simulink model "QiMotorController_ModelReference"  (R2021b)
settings: Solver=FixedStepDiscrete  StartTime=0.0  StopTime=5  RelTol=1e-3
PreLoadFcn:
  | RTWConfigurationCB('preloadfcn', bdroot);
PostLoadFcn:
  | load('configuration/data_struct.mat');
  | load('configuration/fluxMaps_propMotor.mat');
  | load('configuration/parameterInit_PROP.mat');
  | load('configuration/parameterInit_PUMP.mat');
  | load('configuration/parameterInit_PITCH.mat');
  | load('configuration/parameterInit_TILT.mat');
  | %load('configuration/base_workspace_signal_definition.mat');
  | %load('resolvedatastores_to_baseworkspace_for_faster_simulation.mat');
model workspace (MAT data in the model file):
  ADC_CALIBRATION_SAMPLES : Simulink.Parameter (value not decoded)
  DEFAULT_RESOLVER_CONTROL_WORD : Simulink.Parameter (value not decoded)
  PLL_FREQUENCY : Simulink.Parameter (value not decoded)
  SIMULATION_OPTIONS : Simulink.Parameter (value not decoded)
  TARGET_CODE_GEN : Simulink.Parameter (value not decoded)
  Ts = 2.5e-07
symbols that are objects in the model workspace (value not decoded): PLL_FREQUENCY, TARGET_CODE_GEN
undefined symbols (not defined in the file): DEADTIME_NS__PITCH, DEADTIME_NS__PROP, DEADTIME_NS__PUMP, DEADTIME_NS__TILT, fIa_, fIb_, fIc_, fIdc_, fMotorEncoderFloat_, fMotorSensorSpeed_, fUa_, fUb_, fUc_, fUdc_, inbtilt, mdl_pitch_uiAPUFlags, mdl_pitch_uiFlags, modelData, oMot_, oOut_, opInputResolverData_, oPitch, oState_, PLANT_SPEED_QUADRATIC_COEFF__PUMP, POLE_PAIRS_INIT__PITCH, POLE_PAIRS_INIT__PROP, POLE_PAIRS_INIT__PUMP, POLE_PAIRS_INIT__TILT, PWM_FREQ_KHZ__PITCH, PWM_FREQ_KHZ__PROP, PWM_FREQ_KHZ__PUMP, R_PHASE_INIT__PITCH, R_PHASE_INIT__PROP, R_PHASE_INIT__TILT, R_PHASE_INIT_PLANT__PUMP, uiControlReadback_, uiGateDriverStatus_
libraries: simulink x51, spsSeriesRLCBranchLib x25, spsMosfetLib x24, powerlib_extras x24, spsCurrentMeasurementLib x17, spsVoltageMeasurementLib x17, spsPermanentMagnetSynchronousMachineLib x3, spsDCVoltageSourceLib x2, motorModelLibrary x2, slpidlib x2, cstblocks x1, spspowerguiLib x1
(part 4 of 5)

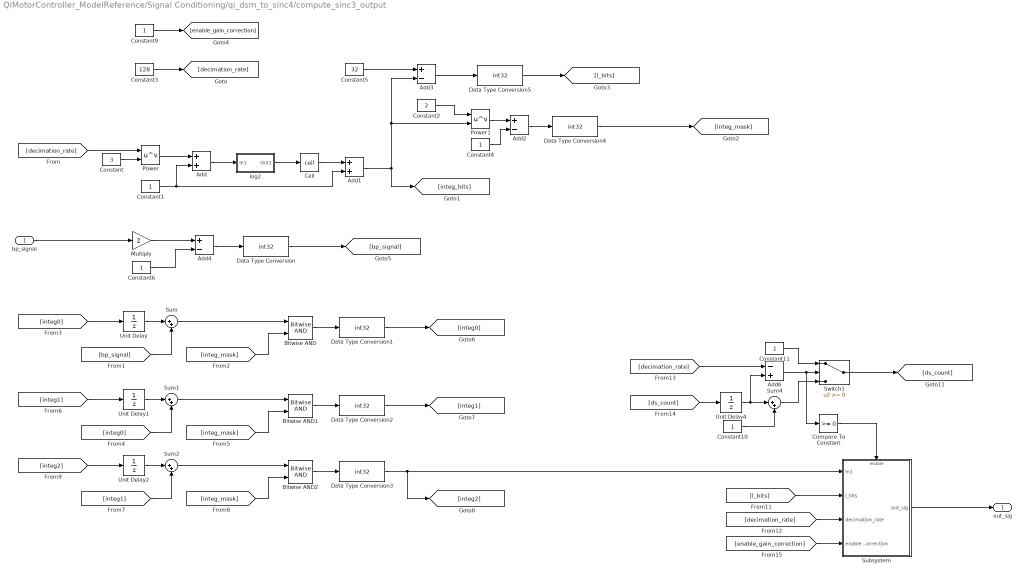
== system QiMotorController_ModelReference/Signal Conditioning/qi_dsm_to_sinc4/compute_sinc3_output ==
  bp_signal : Inport
  Add : Sum
  Add1 : Sum
  Add2 : Sum  Inputs=+-
  Add3 : Sum  Inputs=+-
  Add4 : Sum  Inputs=+-  OutDataTypeStr=int32
  Add6 : Sum  Inputs=-+  OutDataTypeStr=int32
  Bitwise AND : simulink/Logic and Bit Operations/Bitwise Operator  logicop=AND  UseBitMask=off  NumInputPorts=2  BitMask=bin2dec('11011001')  BitMaskRealWorld=Stored Integer
  Bitwise AND1 : simulink/Logic and Bit Operations/Bitwise Operator  logicop=AND  UseBitMask=off  NumInputPorts=2  BitMask=bin2dec('11011001')  BitMaskRealWorld=Stored Integer
  Bitwise AND2 : simulink/Logic and Bit Operations/Bitwise Operator  logicop=AND  UseBitMask=off  NumInputPorts=2  BitMask=bin2dec('11011001')  BitMaskRealWorld=Stored Integer
  Ceil : Rounding  Operator=ceil
  Compare To Constant : simulink/Logic and Bit Operations/Compare To Constant  relop=>=  const=0  OutDataTypeStr=boolean
  Constant : Constant  Value=3  OutDataTypeStr=single  SampleTime=-1
  Constant1 : Constant  OutDataTypeStr=single  SampleTime=-1
  Constant10 : Constant  OutDataTypeStr=int32  SampleTime=-1
  Constant11 : Constant  OutDataTypeStr=int32  SampleTime=-1
  Constant2 : Constant  Value=2  OutDataTypeStr=single  SampleTime=-1
  Constant3 : Constant  Value=128  OutDataTypeStr=single  SampleTime=-1
  Constant4 : Constant  OutDataTypeStr=single  SampleTime=-1
  Constant5 : Constant  Value=32  OutDataTypeStr=single  SampleTime=-1
  Constant6 : Constant  OutDataTypeStr=single  SampleTime=-1
  Constant9 : Constant  OutDataTypeStr=boolean  SampleTime=-1
  Data Type Conversion{,1..5} (6 alike) : DataTypeConversion  OutDataTypeStr=int32
  Multiply : Gain  Gain=2
  Power : Math  Operator=pow  SaturateOnIntegerOverflow=on
  Power1 : Math  Operator=pow  SaturateOnIntegerOverflow=on
  Subsystem : Subsystem
  Sum{,1..2,4} (4 alike) : Sum  Inputs=|++
  Switch1 : Switch
  Unit Delay : UnitDelay  SampleTime=-1  HasFrameUpgradeWarning=on
  Unit Delay1 : UnitDelay  SampleTime=-1  HasFrameUpgradeWarning=on
  Unit Delay2 : UnitDelay  SampleTime=-1  HasFrameUpgradeWarning=on
  Unit Delay4 : UnitDelay  InitialCondition=1  SampleTime=-1  HasFrameUpgradeWarning=on
  log2 : Subsystem
  out_sig : Outport
  wires:
  [decimation_rate] -> Power/1
  Constant/1 -> Power/2
  Power/1 -> Add/1
  Constant1/1 -> Add1/2, Add/2
  Constant3/1 -> [decimation_rate]
  Add/1 -> log2/1(In1)
  log2/1(Out1) -> Ceil/1
  Ceil/1 -> Add1/1
  Add1/1 -> Add3/2, Power1/2, [integ_bits]
  Constant2/1 -> Power1/1
  Power1/1 -> Add2/1
  Constant4/1 -> Add2/2
  Add2/1 -> Data Type Conversion4/1
  Constant5/1 -> Add3/1
  Add3/1 -> Data Type Conversion5/1
  bp_signal/1 -> Multiply/1
  Multiply/1 -> Add4/1
  Constant6/1 -> Add4/2
  Add4/1 -> Data Type Conversion/1
  Data Type Conversion/1 -> [bp_signal]
  Sum/1 -> Bitwise AND/1
  Unit Delay/1 -> Sum/1
  [bp_signal] -> Sum/2
  [integ_mask] -> Bitwise AND/2
  Bitwise AND/1 -> Data Type Conversion1/1
  Data Type Conversion1/1 -> [integ0]
  [integ0] -> Unit Delay/1
  Bitwise AND1/1 -> Data Type Conversion2/1
  [integ1] -> Unit Delay1/1
  [integ_mask] -> Bitwise AND1/2
  Unit Delay1/1 -> Sum1/1
  Sum1/1 -> Bitwise AND1/1
  [integ0] -> Sum1/2
  Unit Delay2/1 -> Sum2/1
  Bitwise AND2/1 -> Data Type Conversion3/1
  [integ1] -> Sum2/2
  [integ2] -> Unit Delay2/1
  Sum2/1 -> Bitwise AND2/1
  [integ_mask] -> Bitwise AND2/2
  Data Type Conversion4/1 -> [integ_mask]
  Data Type Conversion5/1 -> [l_bits]
  Constant9/1 -> [enable_gain_correction]
  Subsystem/1(out_sig) -> out_sig/1
  Sum4/1 -> Switch1/3
  Constant10/1 -> Sum4/2
  Unit Delay4/1 -> Sum4/1, Add6/2
  Constant11/1 -> Switch1/1
  Switch1/1 -> [ds_count]
  [ds_count] -> Unit Delay4/1
  [decimation_rate] -> Add6/1
  Add6/1 -> Compare To Constant/1, Switch1/2
  Compare To Constant/1 -> Subsystem/Enable
  Data Type Conversion3/1 -> [integ2], Subsystem/1(In1)
  Data Type Conversion2/1 -> [integ1]
  [l_bits] -> Subsystem/2(l_bits)
  [decimation_rate] -> Subsystem/3(decimation_rate)
  [enable_gain_correction] -> Subsystem/4(enable_gain_correction)

== system QiMotorController_ModelReference/Signal Conditioning/qi_dsm_to_sinc5/compute_dsm_output ==
  sig_in : Inport
  Add : Sum  Inputs=+-
  Add{1,3..7} (6 alike) : Sum
  Add2 : Sum  Inputs=+-
  Compare To Constant : simulink/Logic and Bit Operations/Compare To Constant  relop=>=  const=0  OutDataTypeStr=boolean
  Constant : Constant  SampleTime=-1
  Constant1 : Constant  Value=0  SampleTime=-1
  Constant2 : Constant  SampleTime=-1
  Constant3 : Constant  Value=2  SampleTime=-1
  Divide{,1..7} (8 alike) : Product  Inputs=**
  Switch : Switch  Criteria=u2 > Threshold
  Switch1 : Switch  Criteria=u2 > Threshold
  Switch2 : Switch  Criteria=u2 > Threshold
  Unit Delay{,1..6} (7 alike) : UnitDelay  SampleTime=-1  HasFrameUpgradeWarning=on
  pdm_signal : Outport
  wires:
  [b2] -> Divide/1
  [vref] -> Divide/2
  [s1_accum] -> Unit Delay1/1
  Divide/1 -> Add/2
  [s2_accum] -> Unit Delay/1
  [a2] -> Divide1/1
  Add/1 -> Divide1/2
  Unit Delay1/1 -> Add/1
  Unit Delay/1 -> Add1/1
  Divide1/1 -> Add1/2
  [vref] -> Divide2/2
  [b1] -> Divide2/1
  Divide2/1 -> Add2/2
  [a1] -> Divide3/1
  Add2/1 -> Divide3/2
  [s1_accum] -> Unit Delay2/1
  Unit Delay2/1 -> Add3/1
  Divide3/1 -> Add3/2
  [s2_accum] -> Unit Delay3/1
  Unit Delay3/1 -> Compare To Constant/1
  Add1/1 -> Switch/1
  Add3/1 -> Switch1/1
  Switch1/1 -> [s1_accum]
  Switch/1 -> [s2_accum]
  Compare To Constant/1 -> Switch1/2, Switch/2, Switch2/2
  Switch2/1 -> [dout], pdm_signal/1
  Constant/1 -> Switch2/1
  Constant1/1 -> Switch2/3
  [s2_accum] -> Unit Delay4/1
  Unit Delay4/1 -> Add5/1
  [s1_accum] -> Unit Delay5/1
  [a2] -> Divide5/1
  [vref] -> Divide4/2
  Add4/1 -> Divide5/2
  Unit Delay5/1 -> Add4/1
  [b2] -> Divide4/1
  Add5/1 -> Switch/3
  Divide5/1 -> Add5/2
  Divide4/1 -> Add4/2
  [s1_accum] -> Unit Delay6/1
  [b1] -> Divide6/1
  Divide7/1 -> Add7/2
  Add7/1 -> Switch1/3
  [a1] -> Divide7/1
  sig_in/1 -> Add6/1, Add2/1
  Add6/1 -> Divide7/2
  Unit Delay6/1 -> Add7/1
  [vref] -> Divide6/2
  Divide6/1 -> Add6/2
  Constant2/1 -> [a2], [vref], [b1], [a1]
  Constant3/1 -> [b2]

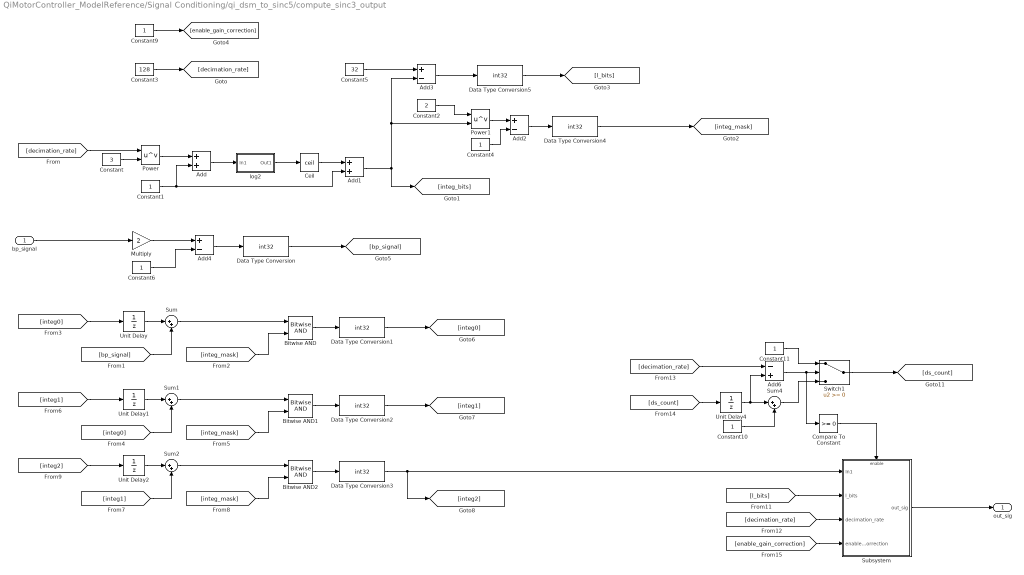
== system QiMotorController_ModelReference/Signal Conditioning/qi_dsm_to_sinc5/compute_sinc3_output ==
  bp_signal : Inport
  Add : Sum
  Add1 : Sum
  Add2 : Sum  Inputs=+-
  Add3 : Sum  Inputs=+-
  Add4 : Sum  Inputs=+-  OutDataTypeStr=int32
  Add6 : Sum  Inputs=-+  OutDataTypeStr=int32
  Bitwise AND : simulink/Logic and Bit Operations/Bitwise Operator  logicop=AND  UseBitMask=off  NumInputPorts=2  BitMask=bin2dec('11011001')  BitMaskRealWorld=Stored Integer
  Bitwise AND1 : simulink/Logic and Bit Operations/Bitwise Operator  logicop=AND  UseBitMask=off  NumInputPorts=2  BitMask=bin2dec('11011001')  BitMaskRealWorld=Stored Integer
  Bitwise AND2 : simulink/Logic and Bit Operations/Bitwise Operator  logicop=AND  UseBitMask=off  NumInputPorts=2  BitMask=bin2dec('11011001')  BitMaskRealWorld=Stored Integer
  Ceil : Rounding  Operator=ceil
  Compare To Constant : simulink/Logic and Bit Operations/Compare To Constant  relop=>=  const=0  OutDataTypeStr=boolean
  Constant : Constant  Value=3  OutDataTypeStr=single  SampleTime=-1
  Constant1 : Constant  OutDataTypeStr=single  SampleTime=-1
  Constant10 : Constant  OutDataTypeStr=int32  SampleTime=-1
  Constant11 : Constant  OutDataTypeStr=int32  SampleTime=-1
  Constant2 : Constant  Value=2  OutDataTypeStr=single  SampleTime=-1
  Constant3 : Constant  Value=128  OutDataTypeStr=single  SampleTime=-1
  Constant4 : Constant  OutDataTypeStr=single  SampleTime=-1
  Constant5 : Constant  Value=32  OutDataTypeStr=single  SampleTime=-1
  Constant6 : Constant  OutDataTypeStr=single  SampleTime=-1
  Constant9 : Constant  OutDataTypeStr=boolean  SampleTime=-1
  Data Type Conversion{,1..5} (6 alike) : DataTypeConversion  OutDataTypeStr=int32
  Multiply : Gain  Gain=2
  Power : Math  Operator=pow  SaturateOnIntegerOverflow=on
  Power1 : Math  Operator=pow  SaturateOnIntegerOverflow=on
  Subsystem : Subsystem
  Sum{,1..2,4} (4 alike) : Sum  Inputs=|++
  Switch1 : Switch
  Unit Delay : UnitDelay  SampleTime=-1  HasFrameUpgradeWarning=on
  Unit Delay1 : UnitDelay  SampleTime=-1  HasFrameUpgradeWarning=on
  Unit Delay2 : UnitDelay  SampleTime=-1  HasFrameUpgradeWarning=on
  Unit Delay4 : UnitDelay  InitialCondition=1  SampleTime=-1  HasFrameUpgradeWarning=on
  log2 : Subsystem
  out_sig : Outport
  wires:
  [decimation_rate] -> Power/1
  Constant/1 -> Power/2
  Power/1 -> Add/1
  Constant1/1 -> Add1/2, Add/2
  Constant3/1 -> [decimation_rate]
  Add/1 -> log2/1(In1)
  log2/1(Out1) -> Ceil/1
  Ceil/1 -> Add1/1
  Add1/1 -> Add3/2, Power1/2, [integ_bits]
  Constant2/1 -> Power1/1
  Power1/1 -> Add2/1
  Constant4/1 -> Add2/2
  Add2/1 -> Data Type Conversion4/1
  Constant5/1 -> Add3/1
  Add3/1 -> Data Type Conversion5/1
  bp_signal/1 -> Multiply/1
  Multiply/1 -> Add4/1
  Constant6/1 -> Add4/2
  Add4/1 -> Data Type Conversion/1
  Data Type Conversion/1 -> [bp_signal]
  Sum/1 -> Bitwise AND/1
  Unit Delay/1 -> Sum/1
  [bp_signal] -> Sum/2
  [integ_mask] -> Bitwise AND/2
  Bitwise AND/1 -> Data Type Conversion1/1
  Data Type Conversion1/1 -> [integ0]
  [integ0] -> Unit Delay/1
  Bitwise AND1/1 -> Data Type Conversion2/1
  [integ1] -> Unit Delay1/1
  [integ_mask] -> Bitwise AND1/2
  Unit Delay1/1 -> Sum1/1
  Sum1/1 -> Bitwise AND1/1
  [integ0] -> Sum1/2
  Unit Delay2/1 -> Sum2/1
  Bitwise AND2/1 -> Data Type Conversion3/1
  [integ1] -> Sum2/2
  [integ2] -> Unit Delay2/1
  Sum2/1 -> Bitwise AND2/1
  [integ_mask] -> Bitwise AND2/2
  Data Type Conversion4/1 -> [integ_mask]
  Data Type Conversion5/1 -> [l_bits]
  Constant9/1 -> [enable_gain_correction]
  Subsystem/1(out_sig) -> out_sig/1
  Sum4/1 -> Switch1/3
  Constant10/1 -> Sum4/2
  Unit Delay4/1 -> Sum4/1, Add6/2
  Constant11/1 -> Switch1/1
  Switch1/1 -> [ds_count]
  [ds_count] -> Unit Delay4/1
  [decimation_rate] -> Add6/1
  Add6/1 -> Compare To Constant/1, Switch1/2
  Compare To Constant/1 -> Subsystem/Enable
  Data Type Conversion3/1 -> [integ2], Subsystem/1(In1)
  Data Type Conversion2/1 -> [integ1]
  [l_bits] -> Subsystem/2(l_bits)
  [decimation_rate] -> Subsystem/3(decimation_rate)
  [enable_gain_correction] -> Subsystem/4(enable_gain_correction)

== system QiMotorController_ModelReference/Signal Conditioning/qi_dsm_to_sinc6/compute_dsm_output ==
  sig_in : Inport
  Add : Sum  Inputs=+-
  Add{1,3..7} (6 alike) : Sum
  Add2 : Sum  Inputs=+-
  Compare To Constant : simulink/Logic and Bit Operations/Compare To Constant  relop=>=  const=0  OutDataTypeStr=boolean
  Constant : Constant  SampleTime=-1
  Constant1 : Constant  Value=0  SampleTime=-1
  Constant2 : Constant  SampleTime=-1
  Constant3 : Constant  Value=2  SampleTime=-1
  Divide{,1..7} (8 alike) : Product  Inputs=**
  Switch : Switch  Criteria=u2 > Threshold
  Switch1 : Switch  Criteria=u2 > Threshold
  Switch2 : Switch  Criteria=u2 > Threshold
  Unit Delay{,1..6} (7 alike) : UnitDelay  SampleTime=-1  HasFrameUpgradeWarning=on
  pdm_signal : Outport
  wires:
  [b2] -> Divide/1
  [vref] -> Divide/2
  [s1_accum] -> Unit Delay1/1
  Divide/1 -> Add/2
  [s2_accum] -> Unit Delay/1
  [a2] -> Divide1/1
  Add/1 -> Divide1/2
  Unit Delay1/1 -> Add/1
  Unit Delay/1 -> Add1/1
  Divide1/1 -> Add1/2
  [vref] -> Divide2/2
  [b1] -> Divide2/1
  Divide2/1 -> Add2/2
  [a1] -> Divide3/1
  Add2/1 -> Divide3/2
  [s1_accum] -> Unit Delay2/1
  Unit Delay2/1 -> Add3/1
  Divide3/1 -> Add3/2
  [s2_accum] -> Unit Delay3/1
  Unit Delay3/1 -> Compare To Constant/1
  Add1/1 -> Switch/1
  Add3/1 -> Switch1/1
  Switch1/1 -> [s1_accum]
  Switch/1 -> [s2_accum]
  Compare To Constant/1 -> Switch1/2, Switch/2, Switch2/2
  Switch2/1 -> [dout], pdm_signal/1
  Constant/1 -> Switch2/1
  Constant1/1 -> Switch2/3
  [s2_accum] -> Unit Delay4/1
  Unit Delay4/1 -> Add5/1
  [s1_accum] -> Unit Delay5/1
  [a2] -> Divide5/1
  [vref] -> Divide4/2
  Add4/1 -> Divide5/2
  Unit Delay5/1 -> Add4/1
  [b2] -> Divide4/1
  Add5/1 -> Switch/3
  Divide5/1 -> Add5/2
  Divide4/1 -> Add4/2
  [s1_accum] -> Unit Delay6/1
  [b1] -> Divide6/1
  Divide7/1 -> Add7/2
  Add7/1 -> Switch1/3
  [a1] -> Divide7/1
  sig_in/1 -> Add6/1, Add2/1
  Add6/1 -> Divide7/2
  Unit Delay6/1 -> Add7/1
  [vref] -> Divide6/2
  Divide6/1 -> Add6/2
  Constant2/1 -> [a2], [vref], [b1], [a1]
  Constant3/1 -> [b2]

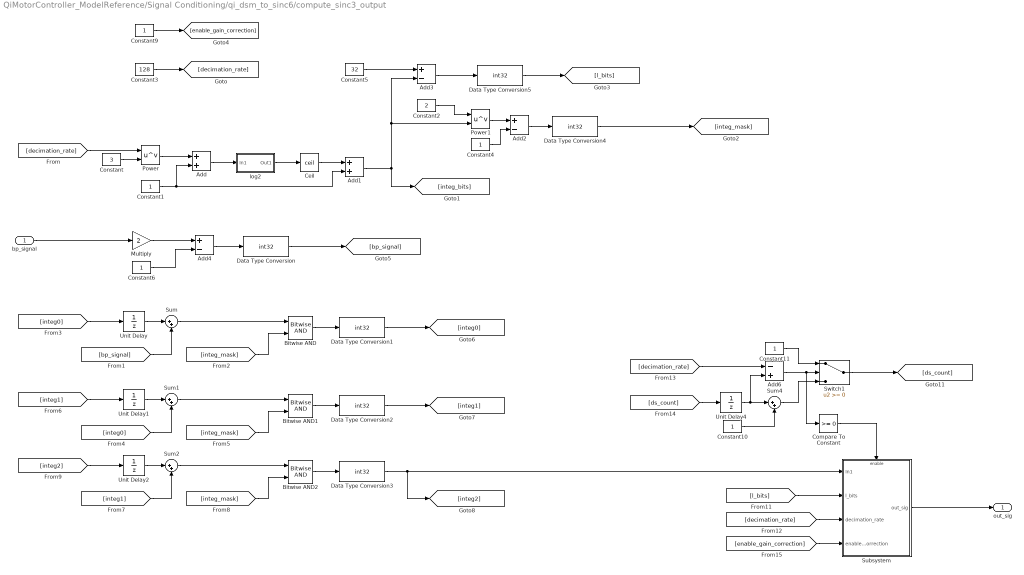
== system QiMotorController_ModelReference/Signal Conditioning/qi_dsm_to_sinc6/compute_sinc3_output ==
  bp_signal : Inport
  Add : Sum
  Add1 : Sum
  Add2 : Sum  Inputs=+-
  Add3 : Sum  Inputs=+-
  Add4 : Sum  Inputs=+-  OutDataTypeStr=int32
  Add6 : Sum  Inputs=-+  OutDataTypeStr=int32
  Bitwise AND : simulink/Logic and Bit Operations/Bitwise Operator  logicop=AND  UseBitMask=off  NumInputPorts=2  BitMask=bin2dec('11011001')  BitMaskRealWorld=Stored Integer
  Bitwise AND1 : simulink/Logic and Bit Operations/Bitwise Operator  logicop=AND  UseBitMask=off  NumInputPorts=2  BitMask=bin2dec('11011001')  BitMaskRealWorld=Stored Integer
  Bitwise AND2 : simulink/Logic and Bit Operations/Bitwise Operator  logicop=AND  UseBitMask=off  NumInputPorts=2  BitMask=bin2dec('11011001')  BitMaskRealWorld=Stored Integer
  Ceil : Rounding  Operator=ceil
  Compare To Constant : simulink/Logic and Bit Operations/Compare To Constant  relop=>=  const=0  OutDataTypeStr=boolean
  Constant : Constant  Value=3  OutDataTypeStr=single  SampleTime=-1
  Constant1 : Constant  OutDataTypeStr=single  SampleTime=-1
  Constant10 : Constant  OutDataTypeStr=int32  SampleTime=-1
  Constant11 : Constant  OutDataTypeStr=int32  SampleTime=-1
  Constant2 : Constant  Value=2  OutDataTypeStr=single  SampleTime=-1
  Constant3 : Constant  Value=128  OutDataTypeStr=single  SampleTime=-1
  Constant4 : Constant  OutDataTypeStr=single  SampleTime=-1
  Constant5 : Constant  Value=32  OutDataTypeStr=single  SampleTime=-1
  Constant6 : Constant  OutDataTypeStr=single  SampleTime=-1
  Constant9 : Constant  OutDataTypeStr=boolean  SampleTime=-1
  Data Type Conversion{,1..5} (6 alike) : DataTypeConversion  OutDataTypeStr=int32
  Multiply : Gain  Gain=2
  Power : Math  Operator=pow  SaturateOnIntegerOverflow=on
  Power1 : Math  Operator=pow  SaturateOnIntegerOverflow=on
  Subsystem : Subsystem
  Sum{,1..2,4} (4 alike) : Sum  Inputs=|++
  Switch1 : Switch
  Unit Delay : UnitDelay  SampleTime=-1  HasFrameUpgradeWarning=on
  Unit Delay1 : UnitDelay  SampleTime=-1  HasFrameUpgradeWarning=on
  Unit Delay2 : UnitDelay  SampleTime=-1  HasFrameUpgradeWarning=on
  Unit Delay4 : UnitDelay  InitialCondition=1  SampleTime=-1  HasFrameUpgradeWarning=on
  log2 : Subsystem
  out_sig : Outport
  wires:
  [decimation_rate] -> Power/1
  Constant/1 -> Power/2
  Power/1 -> Add/1
  Constant1/1 -> Add1/2, Add/2
  Constant3/1 -> [decimation_rate]
  Add/1 -> log2/1(In1)
  log2/1(Out1) -> Ceil/1
  Ceil/1 -> Add1/1
  Add1/1 -> Add3/2, Power1/2, [integ_bits]
  Constant2/1 -> Power1/1
  Power1/1 -> Add2/1
  Constant4/1 -> Add2/2
  Add2/1 -> Data Type Conversion4/1
  Constant5/1 -> Add3/1
  Add3/1 -> Data Type Conversion5/1
  bp_signal/1 -> Multiply/1
  Multiply/1 -> Add4/1
  Constant6/1 -> Add4/2
  Add4/1 -> Data Type Conversion/1
  Data Type Conversion/1 -> [bp_signal]
  Sum/1 -> Bitwise AND/1
  Unit Delay/1 -> Sum/1
  [bp_signal] -> Sum/2
  [integ_mask] -> Bitwise AND/2
  Bitwise AND/1 -> Data Type Conversion1/1
  Data Type Conversion1/1 -> [integ0]
  [integ0] -> Unit Delay/1
  Bitwise AND1/1 -> Data Type Conversion2/1
  [integ1] -> Unit Delay1/1
  [integ_mask] -> Bitwise AND1/2
  Unit Delay1/1 -> Sum1/1
  Sum1/1 -> Bitwise AND1/1
  [integ0] -> Sum1/2
  Unit Delay2/1 -> Sum2/1
  Bitwise AND2/1 -> Data Type Conversion3/1
  [integ1] -> Sum2/2
  [integ2] -> Unit Delay2/1
  Sum2/1 -> Bitwise AND2/1
  [integ_mask] -> Bitwise AND2/2
  Data Type Conversion4/1 -> [integ_mask]
  Data Type Conversion5/1 -> [l_bits]
  Constant9/1 -> [enable_gain_correction]
  Subsystem/1(out_sig) -> out_sig/1
  Sum4/1 -> Switch1/3
  Constant10/1 -> Sum4/2
  Unit Delay4/1 -> Sum4/1, Add6/2
  Constant11/1 -> Switch1/1
  Switch1/1 -> [ds_count]
  [ds_count] -> Unit Delay4/1
  [decimation_rate] -> Add6/1
  Add6/1 -> Compare To Constant/1, Switch1/2
  Compare To Constant/1 -> Subsystem/Enable
  Data Type Conversion3/1 -> [integ2], Subsystem/1(In1)
  Data Type Conversion2/1 -> [integ1]
  [l_bits] -> Subsystem/2(l_bits)
  [decimation_rate] -> Subsystem/3(decimation_rate)
  [enable_gain_correction] -> Subsystem/4(enable_gain_correction)

== system QiMotorController_ModelReference/Signal Conditioning/qi_dsm_to_sinc7/compute_dsm_output ==
  sig_in : Inport
  Add : Sum  Inputs=+-
  Add{1,3..7} (6 alike) : Sum
  Add2 : Sum  Inputs=+-
  Compare To Constant : simulink/Logic and Bit Operations/Compare To Constant  relop=>=  const=0  OutDataTypeStr=boolean
  Constant : Constant  SampleTime=-1
  Constant1 : Constant  Value=0  SampleTime=-1
  Constant2 : Constant  SampleTime=-1
  Constant3 : Constant  Value=2  SampleTime=-1
  Divide{,1..7} (8 alike) : Product  Inputs=**
  Scope : Scope  NumInputPorts=2
  Switch : Switch  Criteria=u2 > Threshold
  Switch1 : Switch  Criteria=u2 > Threshold
  Switch2 : Switch  Criteria=u2 > Threshold
  Unit Delay{,1..6} (7 alike) : UnitDelay  SampleTime=-1  HasFrameUpgradeWarning=on
  pdm_signal : Outport
  wires:
  [b2] -> Divide/1
  [vref] -> Divide/2
  [s1_accum] -> Unit Delay1/1
  Divide/1 -> Add/2
  [s2_accum] -> Unit Delay/1
  [a2] -> Divide1/1
  Add/1 -> Divide1/2
  Unit Delay1/1 -> Add/1
  Unit Delay/1 -> Add1/1
  Divide1/1 -> Add1/2
  [vref] -> Divide2/2
  [b1] -> Divide2/1
  Divide2/1 -> Add2/2
  [a1] -> Divide3/1
  Add2/1 -> Divide3/2
  [s1_accum] -> Unit Delay2/1
  Unit Delay2/1 -> Add3/1
  Divide3/1 -> Add3/2
  [s2_accum] -> Unit Delay3/1
  Unit Delay3/1 -> Compare To Constant/1
  Add1/1 -> Switch/1
  Add3/1 -> Switch1/1
  Switch1/1 -> Scope/2, [s1_accum]
  Switch/1 -> Scope/1, [s2_accum]
  Compare To Constant/1 -> Switch1/2, Switch/2, Switch2/2
  Switch2/1 -> [dout], pdm_signal/1
  Constant/1 -> Switch2/1
  Constant1/1 -> Switch2/3
  [s2_accum] -> Unit Delay4/1
  Unit Delay4/1 -> Add5/1
  [s1_accum] -> Unit Delay5/1
  [a2] -> Divide5/1
  [vref] -> Divide4/2
  Add4/1 -> Divide5/2
  Unit Delay5/1 -> Add4/1
  [b2] -> Divide4/1
  Add5/1 -> Switch/3
  Divide5/1 -> Add5/2
  Divide4/1 -> Add4/2
  [s1_accum] -> Unit Delay6/1
  [b1] -> Divide6/1
  Divide7/1 -> Add7/2
  Add7/1 -> Switch1/3
  [a1] -> Divide7/1
  sig_in/1 -> Add6/1, Add2/1
  Add6/1 -> Divide7/2
  Unit Delay6/1 -> Add7/1
  [vref] -> Divide6/2
  Divide6/1 -> Add6/2
  Constant2/1 -> [a2], [vref], [b1], [a1]
  Constant3/1 -> [b2]

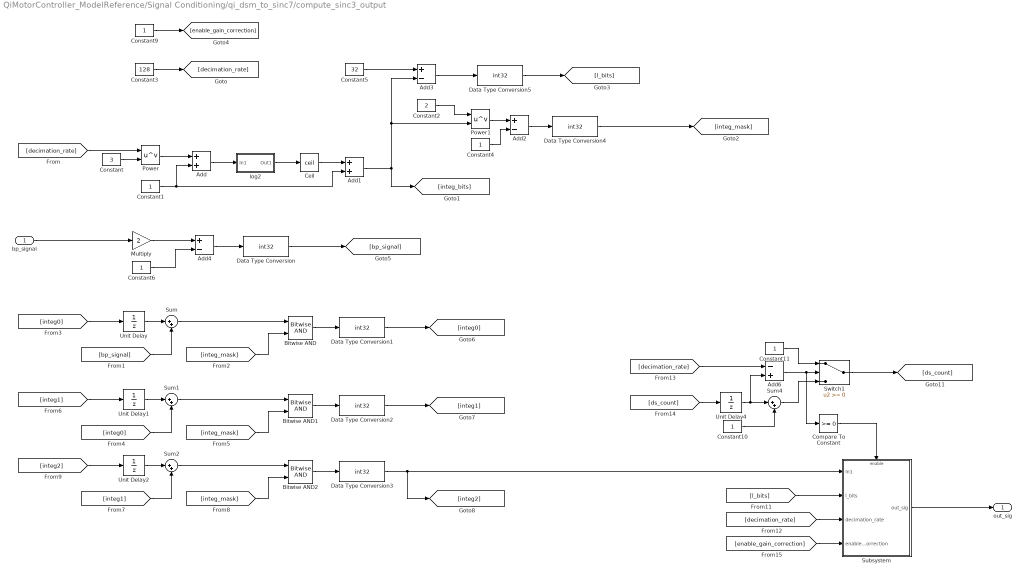
== system QiMotorController_ModelReference/Signal Conditioning/qi_dsm_to_sinc7/compute_sinc3_output ==
  bp_signal : Inport
  Add : Sum
  Add1 : Sum
  Add2 : Sum  Inputs=+-
  Add3 : Sum  Inputs=+-
  Add4 : Sum  Inputs=+-  OutDataTypeStr=int32
  Add6 : Sum  Inputs=-+  OutDataTypeStr=int32
  Bitwise AND : simulink/Logic and Bit Operations/Bitwise Operator  logicop=AND  UseBitMask=off  NumInputPorts=2  BitMask=bin2dec('11011001')  BitMaskRealWorld=Stored Integer
  Bitwise AND1 : simulink/Logic and Bit Operations/Bitwise Operator  logicop=AND  UseBitMask=off  NumInputPorts=2  BitMask=bin2dec('11011001')  BitMaskRealWorld=Stored Integer
  Bitwise AND2 : simulink/Logic and Bit Operations/Bitwise Operator  logicop=AND  UseBitMask=off  NumInputPorts=2  BitMask=bin2dec('11011001')  BitMaskRealWorld=Stored Integer
  Ceil : Rounding  Operator=ceil
  Compare To Constant : simulink/Logic and Bit Operations/Compare To Constant  relop=>=  const=0  OutDataTypeStr=boolean
  Constant : Constant  Value=3  OutDataTypeStr=single  SampleTime=-1
  Constant1 : Constant  OutDataTypeStr=single  SampleTime=-1
  Constant10 : Constant  OutDataTypeStr=int32  SampleTime=-1
  Constant11 : Constant  OutDataTypeStr=int32  SampleTime=-1
  Constant2 : Constant  Value=2  OutDataTypeStr=single  SampleTime=-1
  Constant3 : Constant  Value=128  OutDataTypeStr=single  SampleTime=-1
  Constant4 : Constant  OutDataTypeStr=single  SampleTime=-1
  Constant5 : Constant  Value=32  OutDataTypeStr=single  SampleTime=-1
  Constant6 : Constant  OutDataTypeStr=single  SampleTime=-1
  Constant9 : Constant  OutDataTypeStr=boolean  SampleTime=-1
  Data Type Conversion{,1..5} (6 alike) : DataTypeConversion  OutDataTypeStr=int32
  Multiply : Gain  Gain=2
  Power : Math  Operator=pow  SaturateOnIntegerOverflow=on
  Power1 : Math  Operator=pow  SaturateOnIntegerOverflow=on
  Subsystem : Subsystem
  Sum{,1..2,4} (4 alike) : Sum  Inputs=|++
  Switch1 : Switch
  Unit Delay : UnitDelay  SampleTime=-1  HasFrameUpgradeWarning=on
  Unit Delay1 : UnitDelay  SampleTime=-1  HasFrameUpgradeWarning=on
  Unit Delay2 : UnitDelay  SampleTime=-1  HasFrameUpgradeWarning=on
  Unit Delay4 : UnitDelay  InitialCondition=1  SampleTime=-1  HasFrameUpgradeWarning=on
  log2 : Subsystem
  out_sig : Outport
  wires:
  [decimation_rate] -> Power/1
  Constant/1 -> Power/2
  Power/1 -> Add/1
  Constant1/1 -> Add1/2, Add/2
  Constant3/1 -> [decimation_rate]
  Add/1 -> log2/1(In1)
  log2/1(Out1) -> Ceil/1
  Ceil/1 -> Add1/1
  Add1/1 -> Add3/2, Power1/2, [integ_bits]
  Constant2/1 -> Power1/1
  Power1/1 -> Add2/1
  Constant4/1 -> Add2/2
  Add2/1 -> Data Type Conversion4/1
  Constant5/1 -> Add3/1
  Add3/1 -> Data Type Conversion5/1
  bp_signal/1 -> Multiply/1
  Multiply/1 -> Add4/1
  Constant6/1 -> Add4/2
  Add4/1 -> Data Type Conversion/1
  Data Type Conversion/1 -> [bp_signal]
  Sum/1 -> Bitwise AND/1
  Unit Delay/1 -> Sum/1
  [bp_signal] -> Sum/2
  [integ_mask] -> Bitwise AND/2
  Bitwise AND/1 -> Data Type Conversion1/1
  Data Type Conversion1/1 -> [integ0]
  [integ0] -> Unit Delay/1
  Bitwise AND1/1 -> Data Type Conversion2/1
  [integ1] -> Unit Delay1/1
  [integ_mask] -> Bitwise AND1/2
  Unit Delay1/1 -> Sum1/1
  Sum1/1 -> Bitwise AND1/1
  [integ0] -> Sum1/2
  Unit Delay2/1 -> Sum2/1
  Bitwise AND2/1 -> Data Type Conversion3/1
  [integ1] -> Sum2/2
  [integ2] -> Unit Delay2/1
  Sum2/1 -> Bitwise AND2/1
  [integ_mask] -> Bitwise AND2/2
  Data Type Conversion4/1 -> [integ_mask]
  Data Type Conversion5/1 -> [l_bits]
  Constant9/1 -> [enable_gain_correction]
  Subsystem/1(out_sig) -> out_sig/1
  Sum4/1 -> Switch1/3
  Constant10/1 -> Sum4/2
  Unit Delay4/1 -> Sum4/1, Add6/2
  Constant11/1 -> Switch1/1
  Switch1/1 -> [ds_count]
  [ds_count] -> Unit Delay4/1
  [decimation_rate] -> Add6/1
  Add6/1 -> Compare To Constant/1, Switch1/2
  Compare To Constant/1 -> Subsystem/Enable
  Data Type Conversion3/1 -> [integ2], Subsystem/1(In1)
  Data Type Conversion2/1 -> [integ1]
  [l_bits] -> Subsystem/2(l_bits)
  [decimation_rate] -> Subsystem/3(decimation_rate)
  [enable_gain_correction] -> Subsystem/4(enable_gain_correction)

== system QiMotorController_ModelReference/Signal Conditioning/qi_dsm_to_sinc8/compute_dsm_output ==
  sig_in : Inport
  Add : Sum  Inputs=+-
  Add{1,3..7} (6 alike) : Sum
  Add2 : Sum  Inputs=+-
  Compare To Constant : simulink/Logic and Bit Operations/Compare To Constant  relop=>=  const=0  OutDataTypeStr=boolean
  Constant : Constant  SampleTime=-1
  Constant1 : Constant  Value=0  SampleTime=-1
  Constant2 : Constant  SampleTime=-1
  Constant3 : Constant  Value=2  SampleTime=-1
  Divide{,1..7} (8 alike) : Product  Inputs=**
  Scope : Scope  NumInputPorts=2
  Switch : Switch  Criteria=u2 > Threshold
  Switch1 : Switch  Criteria=u2 > Threshold
  Switch2 : Switch  Criteria=u2 > Threshold
  Unit Delay{,1..6} (7 alike) : UnitDelay  SampleTime=-1  HasFrameUpgradeWarning=on
  pdm_signal : Outport
  wires:
  [b2] -> Divide/1
  [vref] -> Divide/2
  [s1_accum] -> Unit Delay1/1
  Divide/1 -> Add/2
  [s2_accum] -> Unit Delay/1
  [a2] -> Divide1/1
  Add/1 -> Divide1/2
  Unit Delay1/1 -> Add/1
  Unit Delay/1 -> Add1/1
  Divide1/1 -> Add1/2
  [vref] -> Divide2/2
  [b1] -> Divide2/1
  Divide2/1 -> Add2/2
  [a1] -> Divide3/1
  Add2/1 -> Divide3/2
  [s1_accum] -> Unit Delay2/1
  Unit Delay2/1 -> Add3/1
  Divide3/1 -> Add3/2
  [s2_accum] -> Unit Delay3/1
  Unit Delay3/1 -> Compare To Constant/1
  Add1/1 -> Switch/1
  Add3/1 -> Switch1/1
  Switch1/1 -> Scope/2, [s1_accum]
  Switch/1 -> Scope/1, [s2_accum]
  Compare To Constant/1 -> Switch1/2, Switch/2, Switch2/2
  Switch2/1 -> [dout], pdm_signal/1
  Constant/1 -> Switch2/1
  Constant1/1 -> Switch2/3
  [s2_accum] -> Unit Delay4/1
  Unit Delay4/1 -> Add5/1
  [s1_accum] -> Unit Delay5/1
  [a2] -> Divide5/1
  [vref] -> Divide4/2
  Add4/1 -> Divide5/2
  Unit Delay5/1 -> Add4/1
  [b2] -> Divide4/1
  Add5/1 -> Switch/3
  Divide5/1 -> Add5/2
  Divide4/1 -> Add4/2
  [s1_accum] -> Unit Delay6/1
  [b1] -> Divide6/1
  Divide7/1 -> Add7/2
  Add7/1 -> Switch1/3
  [a1] -> Divide7/1
  sig_in/1 -> Add6/1, Add2/1
  Add6/1 -> Divide7/2
  Unit Delay6/1 -> Add7/1
  [vref] -> Divide6/2
  Divide6/1 -> Add6/2
  Constant2/1 -> [a2], [vref], [b1], [a1]
  Constant3/1 -> [b2]

== system QiMotorController_ModelReference/Signal Conditioning/qi_dsm_to_sinc8/compute_sinc3_output ==
  bp_signal : Inport
  Add : Sum
  Add1 : Sum
  Add2 : Sum  Inputs=+-
  Add3 : Sum  Inputs=+-
  Add4 : Sum  Inputs=+-  OutDataTypeStr=int32
  Add6 : Sum  Inputs=-+  OutDataTypeStr=int32
  Bitwise AND : simulink/Logic and Bit Operations/Bitwise Operator  logicop=AND  UseBitMask=off  NumInputPorts=2  BitMask=bin2dec('11011001')  BitMaskRealWorld=Stored Integer
  Bitwise AND1 : simulink/Logic and Bit Operations/Bitwise Operator  logicop=AND  UseBitMask=off  NumInputPorts=2  BitMask=bin2dec('11011001')  BitMaskRealWorld=Stored Integer
  Bitwise AND2 : simulink/Logic and Bit Operations/Bitwise Operator  logicop=AND  UseBitMask=off  NumInputPorts=2  BitMask=bin2dec('11011001')  BitMaskRealWorld=Stored Integer
  Ceil : Rounding  Operator=ceil
  Compare To Constant : simulink/Logic and Bit Operations/Compare To Constant  relop=>=  const=0  OutDataTypeStr=boolean
  Constant : Constant  Value=3  OutDataTypeStr=single  SampleTime=-1
  Constant1 : Constant  OutDataTypeStr=single  SampleTime=-1
  Constant10 : Constant  OutDataTypeStr=int32  SampleTime=-1
  Constant11 : Constant  OutDataTypeStr=int32  SampleTime=-1
  Constant2 : Constant  Value=2  OutDataTypeStr=single  SampleTime=-1
  Constant3 : Constant  Value=128  OutDataTypeStr=single  SampleTime=-1
  Constant4 : Constant  OutDataTypeStr=single  SampleTime=-1
  Constant5 : Constant  Value=32  OutDataTypeStr=single  SampleTime=-1
  Constant6 : Constant  OutDataTypeStr=single  SampleTime=-1
  Constant9 : Constant  OutDataTypeStr=boolean  SampleTime=-1
  Data Type Conversion{,1..5} (6 alike) : DataTypeConversion  OutDataTypeStr=int32
  Multiply : Gain  Gain=2
  Power : Math  Operator=pow  SaturateOnIntegerOverflow=on
  Power1 : Math  Operator=pow  SaturateOnIntegerOverflow=on
  Subsystem : Subsystem
  Sum{,1..2,4} (4 alike) : Sum  Inputs=|++
  Switch1 : Switch
  Unit Delay : UnitDelay  SampleTime=-1  HasFrameUpgradeWarning=on
  Unit Delay1 : UnitDelay  SampleTime=-1  HasFrameUpgradeWarning=on
  Unit Delay2 : UnitDelay  SampleTime=-1  HasFrameUpgradeWarning=on
  Unit Delay4 : UnitDelay  InitialCondition=1  SampleTime=-1  HasFrameUpgradeWarning=on
  log2 : Subsystem
  out_sig : Outport
  wires:
  [decimation_rate] -> Power/1
  Constant/1 -> Power/2
  Power/1 -> Add/1
  Constant1/1 -> Add1/2, Add/2
  Constant3/1 -> [decimation_rate]
  Add/1 -> log2/1(In1)
  log2/1(Out1) -> Ceil/1
  Ceil/1 -> Add1/1
  Add1/1 -> Add3/2, Power1/2, [integ_bits]
  Constant2/1 -> Power1/1
  Power1/1 -> Add2/1
  Constant4/1 -> Add2/2
  Add2/1 -> Data Type Conversion4/1
  Constant5/1 -> Add3/1
  Add3/1 -> Data Type Conversion5/1
  bp_signal/1 -> Multiply/1
  Multiply/1 -> Add4/1
  Constant6/1 -> Add4/2
  Add4/1 -> Data Type Conversion/1
  Data Type Conversion/1 -> [bp_signal]
  Sum/1 -> Bitwise AND/1
  Unit Delay/1 -> Sum/1
  [bp_signal] -> Sum/2
  [integ_mask] -> Bitwise AND/2
  Bitwise AND/1 -> Data Type Conversion1/1
  Data Type Conversion1/1 -> [integ0]
  [integ0] -> Unit Delay/1
  Bitwise AND1/1 -> Data Type Conversion2/1
  [integ1] -> Unit Delay1/1
  [integ_mask] -> Bitwise AND1/2
  Unit Delay1/1 -> Sum1/1
  Sum1/1 -> Bitwise AND1/1
  [integ0] -> Sum1/2
  Unit Delay2/1 -> Sum2/1
  Bitwise AND2/1 -> Data Type Conversion3/1
  [integ1] -> Sum2/2
  [integ2] -> Unit Delay2/1
  Sum2/1 -> Bitwise AND2/1
  [integ_mask] -> Bitwise AND2/2
  Data Type Conversion4/1 -> [integ_mask]
  Data Type Conversion5/1 -> [l_bits]
  Constant9/1 -> [enable_gain_correction]
  Subsystem/1(out_sig) -> out_sig/1
  Sum4/1 -> Switch1/3
  Constant10/1 -> Sum4/2
  Unit Delay4/1 -> Sum4/1, Add6/2
  Constant11/1 -> Switch1/1
  Switch1/1 -> [ds_count]
  [ds_count] -> Unit Delay4/1
  [decimation_rate] -> Add6/1
  Add6/1 -> Compare To Constant/1, Switch1/2
  Compare To Constant/1 -> Subsystem/Enable
  Data Type Conversion3/1 -> [integ2], Subsystem/1(In1)
  Data Type Conversion2/1 -> [integ1]
  [l_bits] -> Subsystem/2(l_bits)
  [decimation_rate] -> Subsystem/3(decimation_rate)
  [enable_gain_correction] -> Subsystem/4(enable_gain_correction)

== system QiMotorController_ModelReference/pitchMotor/PWM_pitch/Center-Aligned PWM 3-Phase   Modulator2 ==
  A_ticks : Inport
  B_ticks : Inport  Port=2
  C_ticks : Inport  Port=3
  Bias : Bias  Bias=1
  Bias1 : Bias  Bias=1
  Bias2 : Bias  Bias=1
  Gain : Gain  Gain=-1
  Gain1 : Gain  Gain=-1
  Gain2 : Gain  Gain=-1
  Mux : Mux  Inputs=6
  Rate Transition1 : RateTransition  Deterministic=off  OutPortSampleTimeOpt=Inherit  OutPortSampleTime=1/PLL_FREQUENCY
  Rate Transition2 : RateTransition  OutPortSampleTime=Ts
  Rate Transition3 : RateTransition  Deterministic=off  OutPortSampleTimeOpt=Inherit  OutPortSampleTime=1/PLL_FREQUENCY
  Rate Transition4 : RateTransition  Deterministic=off  OutPortSampleTimeOpt=Inherit  OutPortSampleTime=1/PLL_FREQUENCY
  Relay : Relay  OnSwitchValue=0  OffSwitchValue=0
  Relay1 : Relay  OnSwitchValue=0  OffSwitchValue=0
  Relay2 : Relay  OnSwitchValue=0  OffSwitchValue=0
  Repeating Sequence : simulink/Sources/Repeating Sequence  rep_seq_t=[0 1/(PWM_FREQ_KHZ__PITCH*1000)/2 1/(PWM_FREQ_KHZ__PITCH*1000)]  rep_seq_y=[0 PLL_FREQUENCY/(PWM_FREQ_KHZ__PITCH*1000)/2 0]
  Scope1 : Scope  NumInputPorts=3
  Scope2 : Scope  NumInputPorts=4
  Sum : Sum  Inputs=|+-
  Sum1 : Sum  Inputs=|+-
  Sum2 : Sum  Inputs=|+-
  PWM Gates : Outport
  wires:
  Rate Transition2/1 -> PWM Gates/1
  Mux/1 -> Rate Transition2/1
  A_ticks/1 -> Rate Transition1/1
  B_ticks/1 -> Rate Transition3/1
  C_ticks/1 -> Rate Transition4/1
  Rate Transition1/1 -> Scope2/2, Sum/1
  Rate Transition3/1 -> Scope2/3, Sum1/1
  Rate Transition4/1 -> Scope2/4, Sum2/1
  Repeating Sequence/1 -> Scope2/1, Sum/2, Sum1/2, Sum2/2
  Sum/1 -> Relay/1
  Sum2/1 -> Relay2/1
  Sum1/1 -> Relay1/1
  Relay1/1 -> Scope1/2, Mux/3, Gain1/1
  Relay2/1 -> Scope1/3, Mux/5, Gain2/1
  Gain1/1 -> Bias/1
  Gain/1 -> Bias1/1
  Gain2/1 -> Bias2/1
  Bias1/1 -> Mux/2
  Bias/1 -> Mux/4
  Bias2/1 -> Mux/6
  Relay/1 -> Gain/1, Scope1/1, Mux/1

== system QiMotorController_ModelReference/propMotor/PWM_prop/Center-Aligned PWM 3-Phase   Modulator1 ==
  Ua : Inport
  Ub : Inport  Port=2
  Uc : Inport  Port=3
  Bias : Bias  Bias=1
  Bias1 : Bias  Bias=1
  Bias2 : Bias  Bias=1
  Gain : Gain  Gain=-1
  Gain1 : Gain  Gain=-1
  Gain2 : Gain  Gain=-1
  Mux : Mux  Inputs=6
  Rate Transition1 : RateTransition  Deterministic=off  OutPortSampleTimeOpt=Inherit  OutPortSampleTime=1/PLL_FREQUENCY
  Rate Transition2 : RateTransition  OutPortSampleTime=Ts
  Rate Transition3 : RateTransition  Deterministic=off  OutPortSampleTimeOpt=Inherit  OutPortSampleTime=1/PLL_FREQUENCY
  Rate Transition4 : RateTransition  Deterministic=off  OutPortSampleTimeOpt=Inherit  OutPortSampleTime=1/PLL_FREQUENCY
  Relay : Relay  OnSwitchValue=0  OffSwitchValue=0
  Relay1 : Relay  OnSwitchValue=0  OffSwitchValue=0
  Relay2 : Relay  OnSwitchValue=0  OffSwitchValue=0
  Repeating Sequence : simulink/Sources/Repeating Sequence  rep_seq_t=[0 1/(PWM_FREQ_KHZ__PROP*1000)/2 1/(PWM_FREQ_KHZ__PROP*1000)]  rep_seq_y=[0 PLL_FREQUENCY/(PWM_FREQ_KHZ__PROP*1000)/2 0]
  Scope1 : Scope  NumInputPorts=3
  Scope2 : Scope
  Sum : Sum  Inputs=|+-
  Sum1 : Sum  Inputs=|+-
  Sum2 : Sum  Inputs=|+-
  PWM Gates : Outport
  wires:
  Rate Transition2/1 -> PWM Gates/1
  Mux/1 -> Rate Transition2/1
  Ua/1 -> Rate Transition1/1
  Ub/1 -> Rate Transition3/1
  Uc/1 -> Rate Transition4/1
  Rate Transition1/1 -> Sum/1
  Rate Transition3/1 -> Sum1/1
  Rate Transition4/1 -> Sum2/1
  Repeating Sequence/1 -> Scope2/1, Sum/2, Sum1/2, Sum2/2
  Sum/1 -> Relay/1
  Sum2/1 -> Relay2/1
  Sum1/1 -> Relay1/1
  Relay1/1 -> Scope1/2, Mux/3, Gain1/1
  Relay2/1 -> Scope1/3, Mux/5, Gain2/1
  Gain1/1 -> Bias/1
  Gain/1 -> Bias1/1
  Gain2/1 -> Bias2/1
  Bias1/1 -> Mux/2
  Bias/1 -> Mux/4
  Bias2/1 -> Mux/6
  Relay/1 -> Gain/1, Scope1/1, Mux/1

== system QiMotorController_ModelReference/propMotor/Sim Option Prop Variant Subsystem/Sim Options 0 Prop Subsystem ==
  In1 : Inport
  600 Nm torque @ 600 rpm1 : Gain  Gain=600/(600/60*2*pi)^2
  Abs1 : Abs
  Add1 : Sum
  Product3 : Product
  Sign1 : Signum
  Square1 : Math  Operator=square  SaturateOnIntegerOverflow=on
  Static friction1 : Constant  Value=10  SampleTime=-1
  Out1 : Outport
  wires:
  600 Nm torque @ 600 rpm1/1 -> Add1/2
  Square1/1 -> 600 Nm torque @ 600 rpm1/1
  Sign1/1 -> Product3/2
  Add1/1 -> Abs1/1
  In1/1 -> Sign1/1, Square1/1
  Static friction1/1 -> Add1/1
  Abs1/1 -> Product3/1
  Product3/1 -> Out1/1  "Torque"

== system QiMotorController_ModelReference/propMotor/Sim Option Prop Variant Subsystem/Sim Options 1 Prop Subsystem ==
  In1 : Inport
  Add2 : Sum  Inputs=-+|
  Constant : Constant  Value=175
  Display1 : Display
  Display2 : Display
  Gain1 : Gain  Gain=-1
  PID Controller : slpidlib/PID Controller  Controller=PI  Form=Parallel  TimeDomain=Discrete-time  UseExternalTs=off  SampleTime=-1  IntegratorMethod=Forward Euler  FilterMethod=Forward Euler  ControllerParametersSource=internal  P=500  I=10000  D=0  UseFilter=on  N=100  TunerSelectOption=Transfer Function Based (PID Tuner App)  InitialConditionSource=internal  InitialConditionForIntegrator=0  InitialConditionForFilter=0  DifferentiatorICPrevScaledInput=0  ExternalReset=none  TrackingMode=off  Kt=1  LimitOutput=on  SatLimitsSource=internal  UpperSaturationLimit=2100  LowerSaturationLimit=-2100  LinearizeAsGain=on  AntiWindupMode=clamping  Kb=1  POutMin=[]  POutMax=[]  IOutMin=[]  IOutMax=[]  DOutMin=[]  DOutMax=[]  NOutMin=[]  NOutMax=[]  SumOutMin=[]  SumOutMax=[]  SaturationOutMin=[]  SaturationOutMax=[]  PParamMin=[]  PParamMax=[]  IParamMin=[]  IParamMax=[]  DParamMin=[]  DParamMax=[]  NParamMin=[]  NParamMax=[]  KbParamMin=[]  KbParamMax=[]  KtParamMin=[]  KtParamMax=[]  KbOutMin=[]  KbOutMax=[]  KtOutMin=[]  KtOutMax=[]  IntegratorOutMin=[]  IntegratorOutMax=[]  FilterOutMin=[]  FilterOutMax=[]  SumI1OutMin=[]  SumI1OutMax=[]  SumI2OutMin=[]  SumI2OutMax=[]  SumI3OutMin=[]  SumI3OutMax=[]  SumI4OutMin=[]  SumI4OutMax=[]  SumDOutMin=[]  SumDOutMax=[]  DifferentiatorOutMin=[]  DifferentiatorOutMax=[]  FilterDiffOutCoefMin=[]  FilterDiffOutCoefMax=[]  ReciprocalOutMin=[]  ReciprocalOutMax=[]  SumDenOutMin=[]  SumDenOutMax=[]  SumNumOutMin=[]  SumNumOutMax=[]  DivideOutMin=[]  DivideOutMax=[]  UdiffTsProdOutMin=[]  UdiffTsProdOutMax=[]  NTsProdOutMin=[]  NTsProdOutMax=[]  UintegralTsProdOutMin=[]  UintegralTsProdOutMax=[]  UngainTsProdOutMin=[]  UngainTsProdOutMax=[]  IntegratorContinuousStateAttributes=''  IntegratorStateMustResolveToSignalObject=off  IntegratorRTWStateStorageClass=Auto  FilterContinuousStateAttributes=''  FilterStateMustResolveToSignalObject=off  FilterRTWStateStorageClass=Auto  ParallelPVariant=InternalParameters  IdealPVariant=Disabled  IVariant=InternalParameters  DVariant=Disabled  IntegratorVariant=Discrete  SatVariant=Enabled  AWVariant=DiscClampingParallel  PCopyVariant=Disabled  TRVariant=Disabled  FdbkBlocksVariant=Forward  IdealPFdbkVariant=Disabled  SatFdbkVariant=Disabled  DerivativeFilterVariant=Disabled  NVariant=Disabled  NCopyVariant=Disabled_SignalSpec  FilterICVariant=Disabled  IntegratorICVariant=InternalICs  ExternalResetVariant=Disabled  TRSumVariant=Passthrough  SumFdbkVariant=Disabled  SumVariant=Sum_PI  TsampFilterVariant=InternalTs  TsampNgainVariant=Passthrough  TsampIntegralVariant=Passthrough  ExternalSaturationOutDataTypeStr=Inherit: Same as second input
  RPM to rad/s2 : Gain  Gain=pi/30
  Out1 : Outport
  wires:
  PID Controller/1 -> Gain1/1
  Add2/1 -> PID Controller/1
  In1/1 -> Add2/1
  RPM to rad/s2/1 -> Display2/1, Add2/2
  Gain1/1 -> Out1/1, Display1/1
  Constant/1 -> RPM to rad/s2/1

== system QiMotorController_ModelReference/pumpfanMotor/PWM_pumpfan/Center-Aligned PWM 3-Phase   Modulator1 ==
  Ua : Inport
  Ub : Inport  Port=2
  Uc : Inport  Port=3
  Bias : Bias  Bias=1
  Bias1 : Bias  Bias=1
  Bias2 : Bias  Bias=1
  Gain : Gain  Gain=-1
  Gain1 : Gain  Gain=-1
  Gain2 : Gain  Gain=-1
  Mux : Mux  Inputs=6
  Rate Transition1 : RateTransition  Deterministic=off  OutPortSampleTimeOpt=Inherit  OutPortSampleTime=1/PLL_FREQUENCY
  Rate Transition2 : RateTransition  OutPortSampleTime=Ts
  Rate Transition3 : RateTransition  Deterministic=off  OutPortSampleTimeOpt=Inherit  OutPortSampleTime=1/PLL_FREQUENCY
  Rate Transition4 : RateTransition  Deterministic=off  OutPortSampleTimeOpt=Inherit  OutPortSampleTime=1/PLL_FREQUENCY
  Relay : Relay  OnSwitchValue=0  OffSwitchValue=0
  Relay1 : Relay  OnSwitchValue=0  OffSwitchValue=0
  Relay2 : Relay  OnSwitchValue=0  OffSwitchValue=0
  Repeating Sequence : simulink/Sources/Repeating Sequence  rep_seq_t=[0 1/(PWM_FREQ_KHZ__PUMP*1000)/2 1/(PWM_FREQ_KHZ__PUMP*1000)]  rep_seq_y=[0 PLL_FREQUENCY/(PWM_FREQ_KHZ__PUMP*1000)/2 0]
  Scope1 : Scope  NumInputPorts=3
  Scope2 : Scope
  Sum : Sum  Inputs=|+-
  Sum1 : Sum  Inputs=|+-
  Sum2 : Sum  Inputs=|+-
  PWM Gates : Outport
  wires:
  Rate Transition2/1 -> PWM Gates/1
  Mux/1 -> Rate Transition2/1
  Ua/1 -> Rate Transition1/1
  Ub/1 -> Rate Transition3/1
  Uc/1 -> Rate Transition4/1
  Rate Transition1/1 -> Sum/1
  Rate Transition3/1 -> Sum1/1
  Rate Transition4/1 -> Sum2/1
  Repeating Sequence/1 -> Scope2/1, Sum/2, Sum1/2, Sum2/2
  Sum/1 -> Relay/1
  Sum2/1 -> Relay2/1
  Sum1/1 -> Relay1/1
  Relay1/1 -> Scope1/2, Mux/3, Gain1/1
  Relay2/1 -> Scope1/3, Mux/5, Gain2/1
  Gain1/1 -> Bias/1
  Gain/1 -> Bias1/1
  Gain2/1 -> Bias2/1
  Bias1/1 -> Mux/2
  Bias/1 -> Mux/4
  Bias2/1 -> Mux/6
  Relay/1 -> Gain/1, Scope1/1, Mux/1

== system QiMotorController_ModelReference/pumpfanMotor/Sim Option Pump Variant Subsystem/Sim Options 0 Pump Subsystem ==
  In1 : Inport
  Affinity Law Tq Coeff: Inboard Fan : Constant  Value=PLANT_SPEED_QUADRATIC_COEFF__PUMP  SampleTime=-1
  Gain : Gain  Gain=1/(2*pi)*60
  Math Function1 : Math  Operator=square  SignedPower=on  SaturateOnIntegerOverflow=on
  Product : Product
  Out1 : Outport
  wires:
  In1/1 -> Gain/1
  Product/1 -> Out1/1  "Torque"
  Math Function1/1 -> Product/1
  Gain/1 -> Math Function1/1
  Affinity Law Tq Coeff: Inboard Fan/1 -> Product/2

== system QiMotorController_ModelReference/pumpfanMotor/Sim Option Pump Variant Subsystem/Sim Options 1 Pump Subsystem ==
  In1 : Inport
  Add2 : Sum  Inputs=-+|
  Display1 : Display
  Gain1 : Gain  Gain=-1
  PID Controller : slpidlib/PID Controller  Controller=PI  Form=Parallel  TimeDomain=Discrete-time  UseExternalTs=off  SampleTime=-1  IntegratorMethod=Forward Euler  FilterMethod=Forward Euler  ControllerParametersSource=internal  P=500  I=10000  D=0  UseFilter=on  N=100  TunerSelectOption=Transfer Function Based (PID Tuner App)  InitialConditionSource=internal  InitialConditionForIntegrator=0  InitialConditionForFilter=0  DifferentiatorICPrevScaledInput=0  ExternalReset=none  TrackingMode=off  Kt=1  LimitOutput=on  SatLimitsSource=internal  UpperSaturationLimit=2100  LowerSaturationLimit=-2100  LinearizeAsGain=on  AntiWindupMode=clamping  Kb=1  POutMin=[]  POutMax=[]  IOutMin=[]  IOutMax=[]  DOutMin=[]  DOutMax=[]  NOutMin=[]  NOutMax=[]  SumOutMin=[]  SumOutMax=[]  SaturationOutMin=[]  SaturationOutMax=[]  PParamMin=[]  PParamMax=[]  IParamMin=[]  IParamMax=[]  DParamMin=[]  DParamMax=[]  NParamMin=[]  NParamMax=[]  KbParamMin=[]  KbParamMax=[]  KtParamMin=[]  KtParamMax=[]  KbOutMin=[]  KbOutMax=[]  KtOutMin=[]  KtOutMax=[]  IntegratorOutMin=[]  IntegratorOutMax=[]  FilterOutMin=[]  FilterOutMax=[]  SumI1OutMin=[]  SumI1OutMax=[]  SumI2OutMin=[]  SumI2OutMax=[]  SumI3OutMin=[]  SumI3OutMax=[]  SumI4OutMin=[]  SumI4OutMax=[]  SumDOutMin=[]  SumDOutMax=[]  DifferentiatorOutMin=[]  DifferentiatorOutMax=[]  FilterDiffOutCoefMin=[]  FilterDiffOutCoefMax=[]  ReciprocalOutMin=[]  ReciprocalOutMax=[]  SumDenOutMin=[]  SumDenOutMax=[]  SumNumOutMin=[]  SumNumOutMax=[]  DivideOutMin=[]  DivideOutMax=[]  UdiffTsProdOutMin=[]  UdiffTsProdOutMax=[]  NTsProdOutMin=[]  NTsProdOutMax=[]  UintegralTsProdOutMin=[]  UintegralTsProdOutMax=[]  UngainTsProdOutMin=[]  UngainTsProdOutMax=[]  IntegratorContinuousStateAttributes=''  IntegratorStateMustResolveToSignalObject=off  IntegratorRTWStateStorageClass=Auto  FilterContinuousStateAttributes=''  FilterStateMustResolveToSignalObject=off  FilterRTWStateStorageClass=Auto  ParallelPVariant=InternalParameters  IdealPVariant=Disabled  IVariant=InternalParameters  DVariant=Disabled  IntegratorVariant=Discrete  SatVariant=Enabled  AWVariant=DiscClampingParallel  PCopyVariant=Disabled  TRVariant=Disabled  FdbkBlocksVariant=Forward  IdealPFdbkVariant=Disabled  SatFdbkVariant=Disabled  DerivativeFilterVariant=Disabled  NVariant=Disabled  NCopyVariant=Disabled_SignalSpec  FilterICVariant=Disabled  IntegratorICVariant=InternalICs  ExternalResetVariant=Disabled  TRSumVariant=Passthrough  SumFdbkVariant=Disabled  SumVariant=Sum_PI  TsampFilterVariant=InternalTs  TsampNgainVariant=Passthrough  TsampIntegralVariant=Passthrough  ExternalSaturationOutDataTypeStr=Inherit: Same as second input
  RPM to rad/s2 : Gain  Gain=pi/30
  Ramp : simulink/Sources/Ramp  slope=4000  start=0  InitialOutput=0
  Out1 : Outport
  wires:
  PID Controller/1 -> Gain1/1
  Add2/1 -> PID Controller/1
  In1/1 -> Add2/1
  RPM to rad/s2/1 -> Add2/2
  Gain1/1 -> Out1/1, Display1/1
  Ramp/1 -> RPM to rad/s2/1

== system QiMotorController_ModelReference/tiltMotor/PWM_tilt/Center-Aligned PWM 3-Phase   Modulator2 ==
  A_ticks : Inport
  B_ticks : Inport  Port=2
  C_ticks : Inport  Port=3
  Bias : Bias  Bias=1
  Bias1 : Bias  Bias=1
  Bias2 : Bias  Bias=1
  Gain : Gain  Gain=-1
  Gain1 : Gain  Gain=-1
  Gain2 : Gain  Gain=-1
  Mux : Mux  Inputs=6
  Rate Transition1 : RateTransition  Deterministic=off  OutPortSampleTimeOpt=Inherit  OutPortSampleTime=1/PLL_FREQUENCY
  Rate Transition2 : RateTransition  OutPortSampleTime=Ts
  Rate Transition3 : RateTransition  Deterministic=off  OutPortSampleTimeOpt=Inherit  OutPortSampleTime=1/PLL_FREQUENCY
  Rate Transition4 : RateTransition  Deterministic=off  OutPortSampleTimeOpt=Inherit  OutPortSampleTime=1/PLL_FREQUENCY
  Relay : Relay  OnSwitchValue=0  OffSwitchValue=0
  Relay1 : Relay  OnSwitchValue=0  OffSwitchValue=0
  Relay2 : Relay  OnSwitchValue=0  OffSwitchValue=0
  Repeating Sequence : simulink/Sources/Repeating Sequence  rep_seq_t=[0 1/(PWM_FREQ_KHZ__PITCH*1000)/2 1/(PWM_FREQ_KHZ__PITCH*1000)]  rep_seq_y=[0 PLL_FREQUENCY/(PWM_FREQ_KHZ__PITCH*1000)/2 0]
  Scope1 : Scope  NumInputPorts=3
  Scope2 : Scope  NumInputPorts=4
  Sum : Sum  Inputs=|+-
  Sum1 : Sum  Inputs=|+-
  Sum2 : Sum  Inputs=|+-
  PWM Gates : Outport
  wires:
  Rate Transition2/1 -> PWM Gates/1
  Mux/1 -> Rate Transition2/1
  A_ticks/1 -> Rate Transition1/1
  B_ticks/1 -> Rate Transition3/1
  C_ticks/1 -> Rate Transition4/1
  Rate Transition1/1 -> Scope2/2, Sum/1
  Rate Transition3/1 -> Scope2/3, Sum1/1
  Rate Transition4/1 -> Scope2/4, Sum2/1
  Repeating Sequence/1 -> Scope2/1, Sum/2, Sum1/2, Sum2/2
  Sum/1 -> Relay/1
  Sum2/1 -> Relay2/1
  Sum1/1 -> Relay1/1
  Relay1/1 -> Scope1/2, Mux/3, Gain1/1
  Relay2/1 -> Scope1/3, Mux/5, Gain2/1
  Gain1/1 -> Bias/1
  Gain/1 -> Bias1/1
  Gain2/1 -> Bias2/1
  Bias1/1 -> Mux/2
  Bias/1 -> Mux/4
  Bias2/1 -> Mux/6
  Relay/1 -> Gain/1, Scope1/1, Mux/1

== system QiMotorController_ModelReference/Fault Injection/pitchMotor_faults/Phase Current & Aux Disturbances/Fault Current Setting ==
  targetPhase : Inport
  Iabc_feedback : Inport  Port=2
  IphMagnitude_value : Inport  Port=3
  Constant : Constant  OutDataTypeStr=uint32  SampleTime=-1
  Constant1 : Constant  Value=2  OutDataTypeStr=uint32  SampleTime=-1
  Constant2 : Constant  Value=3  OutDataTypeStr=uint32  SampleTime=-1
  Constant3 : Constant  Value=0  OutDataTypeStr=single  SampleTime=-1
  Equal : RelationalOperator  Operator===  OutDataTypeStr=boolean  RndMeth=Simplest
  Equal1 : RelationalOperator  Operator===  OutDataTypeStr=boolean  RndMeth=Simplest
  Equal2 : RelationalOperator  Operator===  OutDataTypeStr=boolean  RndMeth=Simplest
  Gain1 : Gain  Gain=-0.5
  GreaterThan : RelationalOperator  Operator=>  OutDataTypeStr=boolean  RndMeth=Simplest
  Mux : Mux  Inputs=3
  Switch{,1..3} (4 alike) : Switch  Criteria=u2 > Threshold
  Iabc_fault : Outport
  wires:
  Constant/1 -> Equal/1
  targetPhase/1 -> Equal/2, Equal2/2, Equal1/2
  Equal/1 -> Switch/2
  Switch/1 -> Mux/1  "Ia_fault"
  Gain1/1 -> Switch2/3, Switch1/3, Switch/3
  Constant1/1 -> Equal1/1
  Equal1/1 -> Switch1/2
  Switch1/1 -> Mux/2  "Ib_fault"
  Equal2/1 -> Switch2/2
  Constant2/1 -> Equal2/1
  Switch2/1 -> Mux/3  "Ic_fault"
  Mux/1 -> Switch3/1
  Constant3/1 -> GreaterThan/2
  IphMagnitude_value/1 -> Switch/1, Switch2/1, Switch1/1, GreaterThan/1, Gain1/1
  GreaterThan/1 -> Switch3/2
  Switch3/1 -> Iabc_fault/1
  Iabc_feedback/1 -> Switch3/3

== system QiMotorController_ModelReference/Fault Injection/pitchMotor_faults/Phase Current & Aux Disturbances/Set uiAPUFlags for Aux Trips ==
  auxTripCode : Inport
  uiAPUFlags : Inport  Port=2
  Constant11 : Constant  OutDataTypeStr=uint32  SampleTime=-1
  Constant12 : Constant  Value=2  OutDataTypeStr=uint32  SampleTime=-1
  Constant13 : Constant  Value=1034  OutDataTypeStr=uint32  SampleTime=-1
  Constant14 : Constant  Value=1035  OutDataTypeStr=uint32  SampleTime=-1
  Equal5 : RelationalOperator  Operator===  OutDataTypeStr=boolean  RndMeth=Simplest
  Equal6 : RelationalOperator  Operator===  OutDataTypeStr=boolean  RndMeth=Simplest
  Switch6 : Switch  Criteria=u2 > Threshold
  Switch7 : Switch  Criteria=u2 > Threshold
  uiAPUFlags_fault : Outport
  wires:
  Constant13/1 -> Equal5/2
  Equal5/1 -> Switch6/2
  Constant11/1 -> Switch6/1
  Constant12/1 -> Switch7/1
  auxTripCode/1 -> Equal5/1, Equal6/1
  Switch7/1 -> Switch6/3
  Equal6/1 -> Switch7/2
  Constant14/1 -> Equal6/2
  uiAPUFlags/1 -> Switch7/3
  Switch6/1 -> uiAPUFlags_fault/1
